simulink model "Prep_Matlab2_P7"  (R2024b)
settings: Solver=VariableStepAuto  StartTime=0.0  StopTime=50  RelTol=1e-3
settings Model: Creator=mikek  LastModifiedBy=keyur

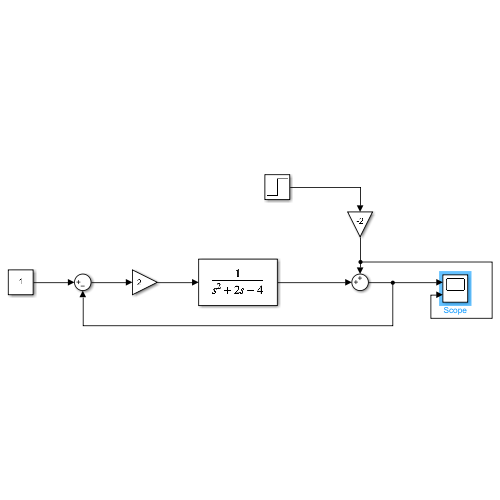
[thumbnail: Simulink's stored preview of the top-level diagram]
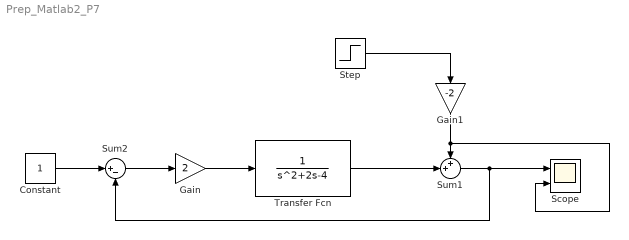
== system Prep_Matlab2_P7 ==
  Constant : Constant
  Gain : Gain  Gain=2
  Gain1 : Gain  Gain=-2
  Scope : Scope  NumInputPorts=2
  Step : Step  Time=15  SampleTime=0
  Sum1 : Sum  Inputs=++|
  Sum2 : Sum  Inputs=|+-
  Transfer Fcn : TransferFcn  Denominator=[1 2 -4]
  wires:
  Sum1/1 -> Sum2/2, Scope/1
  Transfer Fcn/1 -> Sum1/2
  Gain/1 -> Transfer Fcn/1
  Sum2/1 -> Gain/1
  Step/1 -> Gain1/1
  Gain1/1 -> Scope/2, Sum1/1
  Constant/1 -> Sum2/1
